simulink model "UltimoLazoAbiertoCompleto"  (R2023b)
settings: Solver=VariableStepAuto  StartTime=0.0  StopTime=2  FixedStep=0.0005  MaxStep=1e-3  RelTol=1e-3
undefined symbols (not defined in the file or in its folder): alfa, beq, Cts, ee_sli_rtmsupport, g, gcbh, id0, io0, iq0, Jeq, kl, lambda_m, Ld, Lls, Lq, Pp, r, Rs, Rts_amb, tita0, Ts0, wm0
libraries: SignalEditorBlockLib x3, eeTransforms x1, dspsigops x1, spsabctoAlphaBetaZeroLib x1
settings Model: Creator=Gustavo  LastModifiedBy=Gustavo

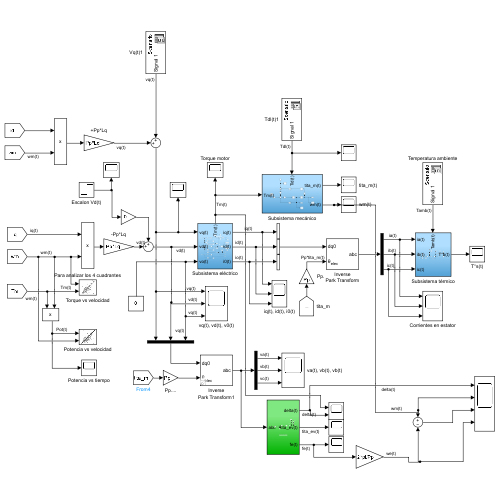
[thumbnail: Simulink's stored preview of the top-level diagram]
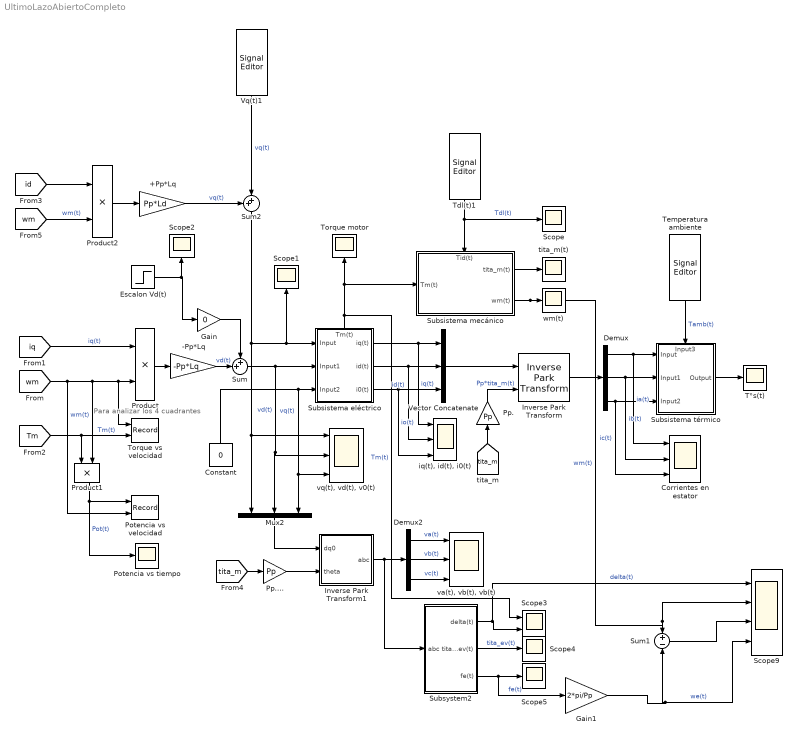
== system UltimoLazoAbiertoCompleto ==
  note: Para analizar los 4 cuadrantes
  +Pp*Lq : Gain  Gain=Pp*Ld
  -Pp*Lq : Gain  Gain=-Pp*Lq
  Constant : Constant  Value=0
  Corrientes en estator : Scope  NumInputPorts=3
  Demux : Demux  Outputs=3
  Demux2 : Demux  Outputs=3
  Escalon Vd(t) : Step  Time=0.5  After=+1.9596  SampleTime=0
  Gain : Gain  Gain=0
  Gain1 : Gain  Gain=2*pi/Pp
  Inverse Park Transform : eeTransforms/Inverse Park Transform  AxisAlignment=Q-axis  PowerInvariant=off
      settings: LibrarySourceBlock=|
      | ee_sl_lib/Mathematical
      | Transforms/Inverse
      | Park Transform
  Inverse Park Transform1 : Subsystem  AncestorBlock=|  LoadFcn=ee_sli_rtmsupport( 'loadfcn', gcbh );  mask(Inverse Park Transform){AxisAlignment=Q-axis, PowerInvariant=off}
      | ee_sl_lib/Mathematical
      | Transforms/Inverse
      | Park Transform
      mask prompts: AxisAlignment "physmod:ee:library:comments:control:eeTransforms:PhaseaAxisAlignment_MP"; PowerInvariant "physmod:ee:library:comments:control:eeTransforms:PowerInvariant_MP"
      mask help: physmod:ee:library:comments:control:eeTransforms:InverseParkTransform_MD
      mask init:
      | if PowerInvariant==0
      |     K1 = 1;
      |     K2 = 1;
      | else
      |     K1 = 1/sqrt(2);
      |     K2 = sqrt(2/3);
      | end
      | 
      | switch AxisAlignment
      |     case 'Q-axis'
      |         Offset = 0;
      |     case 'D-axis'
      |         Offset = pi/2;
      |     otherwise
      | end
      settings: CopyFcn=ee_sli_rtmsupport( 'copyfcn', gcbh );  DeleteFcn=ee_sli_rtmsupport( 'deletefcn', gcbh );  ModelCloseFcn=ee_sli_rtmsupport( 'modelclosefcn', gcbh );  PostSaveFcn=ee_sli_rtmsupport( 'postsavefcn', gcbh );  PreCopyFcn=ee_sli_rtmsupport( 'precopyfcn', gcbh );  OpenFcn=ee_sli_rtmsupport( 'openfcn', gcbh );  CloseFcn=ee_sli_rtmsupport( 'closefcn', gcbh );  PreDeleteFcn=ee_sli_rtmsupport( 'predeletefcn', gcbh );
      settings: LibrarySourceBlock=|
      | ee_sl_lib/Mathematical
      | Transforms/Inverse
      | Park Transform
      mask Help: web(nesl_help(gcbh))
      mask TypeOptions AxisAlignment: physmod:ee:library:comments:control:eeTransforms:Q0x2DAxis_PV | physmod:ee:library:comments:control:eeTransforms:D0x2DAxis_PV
      mask DialogControl AxisAlignment Prompt: Phase-a axis alignment
      mask DialogControl PowerInvariant Prompt: Power invariant
      mask Display: ee.mask.drawInverseParkTransform();
  Mux2 : Mux  Inputs=3
  Potencia vs tiempo : Scope
  Potencia vs velocidad : Record  FileSettingsInternal="{\"entries\":[{\"content\":{\"excelSettings\":{\"content\":{},\"type\":\"Streamout.ExcelSettings\"}},\"type\":\"Streamout.FileSettingStorage\",\"uuid\":\"\"}],\"packageUris\":[\"http:\\/\\/schema.mathworks.com\\/mf0\\/streamout_blocks\\/R2020a\"],\"version\":\"1.0\"}"  Layout=[1 1]  SignalsInternal="{\"entries\":[{\"content\":{\"signals\":[{\"content\":{\"blockPath\":[],\"dimensions\":[1],\"domain\":\"\",\"lineColor\":\"#139fff\",\"port\":1,\"signalID\":16,\"signalName\":\"Pot(t)\"},\"type\":\"RecordBlkView.Signal\",\"uuid\":\"\"},{\"content\":{\"blockPath\":[],\"dimensions\":[1],\"domain\":\"\",\"lineColor\":\"#ff6929\",\"port\":2,\"signalID\":19,\"signalName\":\"wm(t)\"},\"type\":\"RecordBlkView.Signal\",\"uuid\":\"\"}]},\"type\":\"RecordBlkView.InputSignals\",\"uuid\":\"\"}],\"packageUris\":[\"http:\\/\\/schema.mathworks.com\\/mf0\\/streamout_blocks\\/R2020a\"],\"version\":\"1.0\"}"  VisualizationBindings="{\"xyplotplugin\":{\"info\":[{\"series\":[],\"subplotID\":1}]}}"  CompatibilityTag=XY
  Pp. : Gain  Gain=Pp
  Pp.... : Gain  Gain=Pp
  Product : Product
  Product1 : Product
  Product2 : Product
  Scope{,1..2,4..5} (5 alike) : Scope
  Scope3 : Scope  NumInputPorts=2
  Scope9 : Scope  NumInputPorts=4
  Subsistema eléctrico : Subsystem
      settings: PortSchema="{\"entries\":[{\"content\":{\"sides\":[{\"content\":{\"connectorIds\":[\"In1\",\"In2\",\"In3\"]},\"type\":\"ConnectorPlacement.EquallySpacedRectSide\",\"uuid\":\"55314de5-b6ab-4161-b15d-819ac9b3d610\"},{\"content\":{\"connectorIds\":[\"Out1\",\"Out2\",\"Out3\"],\"side\":\"RIGHT\"},\"type\":\"ConnectorPlacement.EquallySpacedRectSide\",\"uuid\":\"6d89c228-26ff-4db5-b942-5bfef0be2fde\"},{\"content\":{\"connectorIds\":[\"Out4\"],\"side\":\"TOP\"},\"type\":\"ConnectorPlacement.EquallySpacedRectSide\",\"uuid\":\"a52f3ca3-a7f6-4886-b92b-9c9e6a107711\"}]},\"type\":\"ConnectorPlacement.EquallySpacedConnector\",\"uuid\":\"22991da4-d60d-4ddc-8bfe-b68e23663f11\"}],\"packageUris\":[\"http://schema.mathworks.com/mf0/Connector/R2020b\"],\"version\":\"1.0\"}"
  Subsistema mecánico : Subsystem
      settings: PortSchema="{\"entries\":[{\"content\":{\"sides\":[{\"content\":{\"connectorIds\":[\"In1\"]},\"type\":\"ConnectorPlacement.EquallySpacedRectSide\",\"uuid\":\"50d48cc3-d7d8-4f90-8b40-173b6a350fbf\"},{\"content\":{\"connectorIds\":[\"Out1\",\"Out2\"],\"side\":\"RIGHT\"},\"type\":\"ConnectorPlacement.EquallySpacedRectSide\",\"uuid\":\"77c04a2b-04e8-45af-8dee-d1b1ab6672f9\"},{\"content\":{\"connectorIds\":[\"In2\"],\"side\":\"TOP\"},\"type\":\"ConnectorPlacement.EquallySpacedRectSide\",\"uuid\":\"9aba66dd-f9d4-41a7-8e04-ce0a031192e2\"}]},\"type\":\"ConnectorPlacement.EquallySpacedConnector\",\"uuid\":\"47c09da0-37f3-4a5d-8fce-2546d5511531\"}],\"packageUris\":[\"http://schema.mathworks.com/mf0/Connector/R2020b\"],\"version\":\"1.0\"}"
  Subsistema térmico : Subsystem
      settings: PortSchema="{\"entries\":[{\"content\":{\"sides\":[{\"content\":{\"connectorIds\":[\"In1\",\"In2\",\"In3\"]},\"type\":\"ConnectorPlacement.EquallySpacedRectSide\",\"uuid\":\"499bb5e3-da94-498d-be5e-1974ba0b4a58\"},{\"content\":{\"connectorIds\":[\"Out1\"],\"side\":\"RIGHT\"},\"type\":\"ConnectorPlacement.EquallySpacedRectSide\",\"uuid\":\"13ea5dea-e51e-4770-b579-88e3e6e50884\"},{\"content\":{\"connectorIds\":[\"In4\"],\"side\":\"TOP\"},\"type\":\"ConnectorPlacement.EquallySpacedRectSide\",\"uuid\":\"72517ed1-a98f-428e-86e2-c370e237c602\"}]},\"type\":\"ConnectorPlacement.EquallySpacedConnector\",\"uuid\":\"7e0eda24-12d6-49d0-ad1f-024c88e78140\"}],\"packageUris\":[\"http://schema.mathworks.com/mf0/Connector/R2020b\"],\"version\":\"1.0\"}"
  Subsystem2 : Subsystem
  Sum : Sum  Inputs=++|
  Sum1 : Sum  Inputs=+|-
  Sum2 : Sum  Inputs=++|
  Tdl(t)1 : SignalEditorBlockLib/Signal Editor  FileName=SeñalTlEstadoInterno.mat  ActiveScenario=Scenario  ActiveSignal=Signal 1  IsBus=off  OutputBusObjectStr=Bus: BusObject  SampleTime=0  Interpolate=off  ZeroCross=off  OutputAfterFinalValue=Setting to zero  Unit=inherit  PreserveSignalName=on  ApplySigPropsToAllScenarios=on  ApplySigPropsToAllSignals=off
  Temperatura ambiente : SignalEditorBlockLib/Signal Editor  FileName=Temperatura ambiente Tamb(t).mat  ActiveScenario=Scenario  ActiveSignal=Signal 1  IsBus=off  OutputBusObjectStr=Bus: BusObject  SampleTime=0  ZeroCross=off  OutputAfterFinalValue=Setting to zero  Unit=inherit  PreserveSignalName=on  ApplySigPropsToAllScenarios=on  ApplySigPropsToAllSignals=off
  Torque motor : Scope
  Torque vs velocidad : Record  FileSettingsInternal="{\"entries\":[{\"content\":{\"excelSettings\":{\"content\":{},\"type\":\"Streamout.ExcelSettings\"}},\"type\":\"Streamout.FileSettingStorage\",\"uuid\":\"\"}],\"packageUris\":[\"http:\\/\\/schema.mathworks.com\\/mf0\\/streamout_blocks\\/R2020a\"],\"version\":\"1.0\"}"  Layout=[1 1]  SignalsInternal="{\"entries\":[{\"content\":{\"signals\":[{\"content\":{\"blockPath\":[],\"dimensions\":[1],\"domain\":\"\",\"lineColor\":\"#64d413\",\"port\":1,\"signalID\":8,\"signalName\":\"wm(t)\"},\"type\":\"RecordBlkView.Signal\",\"uuid\":\"\"},{\"content\":{\"blockPath\":[],\"dimensions\":[1],\"domain\":\"\",\"lineColor\":\"#ff13a6\",\"port\":2,\"signalID\":11,\"signalName\":\"Tm(t)\"},\"type\":\"RecordBlkView.Signal\",\"uuid\":\"\"}]},\"type\":\"RecordBlkView.InputSignals\",\"uuid\":\"\"}],\"packageUris\":[\"http:\\/\\/schema.mathworks.com\\/mf0\\/streamout_blocks\\/R2020a\"],\"version\":\"1.0\"}"  VisualizationBindings="{\"xyplotplugin\":{\"info\":[{\"series\":[],\"subplotID\":1}]}}"  CompatibilityTag=XY
  T°s(t) : Scope
  Vector Concatenate : Concatenate  NumInputs=3
  Vq(t)1 : SignalEditorBlockLib/Signal Editor  FileName=SeñalVQestadoInterno.mat  ActiveScenario=Scenario  ActiveSignal=Signal 1  IsBus=off  OutputBusObjectStr=Bus: BusObject  SampleTime=0  Interpolate=off  ZeroCross=off  OutputAfterFinalValue=Setting to zero  Unit=inherit  PreserveSignalName=on  ApplySigPropsToAllScenarios=on  ApplySigPropsToAllSignals=off
  "iq(t), id(t), i0(t)" : Scope  NumInputPorts=3
  tita_m(t) : Scope
  "va(t), vb(t), vb(t)" : Scope  NumInputPorts=3
  "vq(t), vd(t), v0(t)" : Scope  NumInputPorts=3
  wm(t) : Scope
  wires:
  Tdl(t)1/1 -> Subsistema mecánico/2(Tid(t)), Scope/1  "Tdl(t)"
  Subsistema eléctrico/4(Tm(t)) -> Scope3/1, Subsistema mecánico/1(Tm(t)), Torque motor/1  "Tm(t)"
  Temperatura ambiente/1 -> Subsistema térmico/4(Input3)  "Tamb(t)"
  Subsistema térmico/1(Output) -> T°s(t)/1
  Subsistema eléctrico/2(id(t)) -> "iq(t), id(t), i0(t)"/2, Vector Concatenate/2  "id(t)"
  Subsistema eléctrico/1(iq(t)) -> "iq(t), id(t), i0(t)"/1, Vector Concatenate/1  "iq(t)"
  Demux/2 -> Subsistema térmico/2(Input1), Corrientes en estator/2  "ib(t)"
  Inverse Park Transform/1 -> Demux/1
  Pp./1 -> Inverse Park Transform/2  "Pp*tita_m(t)"
  Subsistema eléctrico/3(i0(t)) -> "iq(t), id(t), i0(t)"/3, Vector Concatenate/3  "io(t)"
  [tita_m] -> Pp./1
  Vector Concatenate/1 -> Inverse Park Transform/1
  Demux/3 -> Subsistema térmico/3(Input2), Corrientes en estator/3  "ic(t)"
  Demux/1 -> Subsistema térmico/1(Input), Corrientes en estator/1  "ia(t)"
  Subsistema mecánico/2(wm(t)) -> Sum1/1, Scope9/2, wm(t)/1  "wm(t)"
  Subsistema mecánico/1(tita_m(t)) -> tita_m(t)/1
  [iq] -> Product/1  "iq(t)"
  Product/1 -> -Pp*Lq/1
  [wm] -> Torque vs velocidad/1, Product/2, Product1/2, Potencia vs velocidad/2  "wm(t)"
  Constant/1 -> Subsistema eléctrico/3(Input2), "vq(t), vd(t), v0(t)"/3, Mux2/3  "vq(t)"
  Inverse Park Transform1/1(abc) -> Subsystem2/1(abc), Demux2/1
  Demux2/1 -> "va(t), vb(t), vb(t)"/1  "va(t)"
  Demux2/3 -> "va(t), vb(t), vb(t)"/3  "vc(t)"
  Demux2/2 -> "va(t), vb(t), vb(t)"/2  "vb(t)"
  [tita_m] -> Pp..../1
  Pp..../1 -> Inverse Park Transform1/2(theta)
  Mux2/1 -> Inverse Park Transform1/1(dq0)
  [Tm] -> Torque vs velocidad/2, Product1/1  "Tm(t)"
  Product1/1 -> Potencia vs tiempo/1, Potencia vs velocidad/1  "Pot(t)"
  Escalon Vd(t)/1 -> Gain/1, Scope2/1
  -Pp*Lq/1 -> Sum/2  "vd(t)"
  Sum/1 -> Subsistema eléctrico/2(Input1), Mux2/2, "vq(t), vd(t), v0(t)"/2  "vd(t)"
  Gain/1 -> Sum/1
  Subsystem2/1(delta(t)) -> Scope9/1, Scope3/2  "delta(t)"
  Subsystem2/2(tita_ev(t)) -> Scope4/1  "tita_ev(t)"
  Subsystem2/3(fe(t)) -> Gain1/1, Scope5/1  "fe(t)"
  Gain1/1 -> Sum1/2, Scope9/4  "we(t)"
  Sum1/1 -> Scope9/3
  Vq(t)1/1 -> Sum2/2  "vq(t)"
  [wm] -> Product2/2  "wm(t)"
  [id] -> Product2/1
  Product2/1 -> +Pp*Lq/1
  +Pp*Lq/1 -> Sum2/1  "vq(t)"
  Sum2/1 -> "vq(t), vd(t), v0(t)"/1, Mux2/1, Scope1/1, Subsistema eléctrico/1(Input)

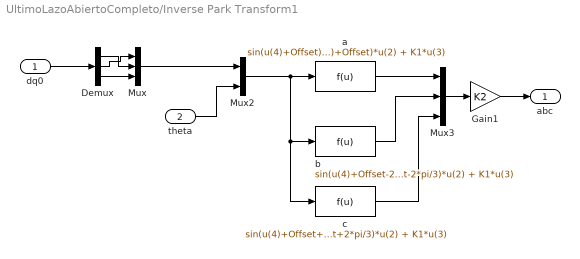
== system UltimoLazoAbiertoCompleto/Inverse Park Transform1 ==
  dq0 : Inport
  theta : Inport  Port=2
  Demux : Demux  Outputs=3
  Gain1 : Gain  Gain=K2
  Mux : Mux  Inputs=3
  Mux2 : Mux  Inputs=2
  Mux3 : Mux  Inputs=3
  a : Fcn  Expr=sin(u(4)+Offset)*u(1) + cos(u(4)+Offset)*u(2) + K1*u(3)
  b : Fcn  Expr=sin(u(4)+Offset-2*pi/3)*u(1) + cos(u(4)+Offset-2*pi/3)*u(2) + K1*u(3)
  c : Fcn  Expr=sin(u(4)+Offset+2*pi/3)*u(1) + cos(u(4)+Offset+2*pi/3)*u(2) + K1*u(3)
  abc : Outport  VectorParamsAs1DForOutWhenUnconnected=off
  wires:
  a/1 -> Mux3/1
  Mux3/1 -> Gain1/1
  Mux2/1 -> a/1, c/1, b/1
  theta/1 -> Mux2/2
  c/1 -> Mux3/3
  Gain1/1 -> abc/1
  b/1 -> Mux3/2
  Demux/2 -> Mux/1
  Demux/1 -> Mux/2
  Demux/3 -> Mux/3
  dq0/1 -> Demux/1
  Mux/1 -> Mux2/1

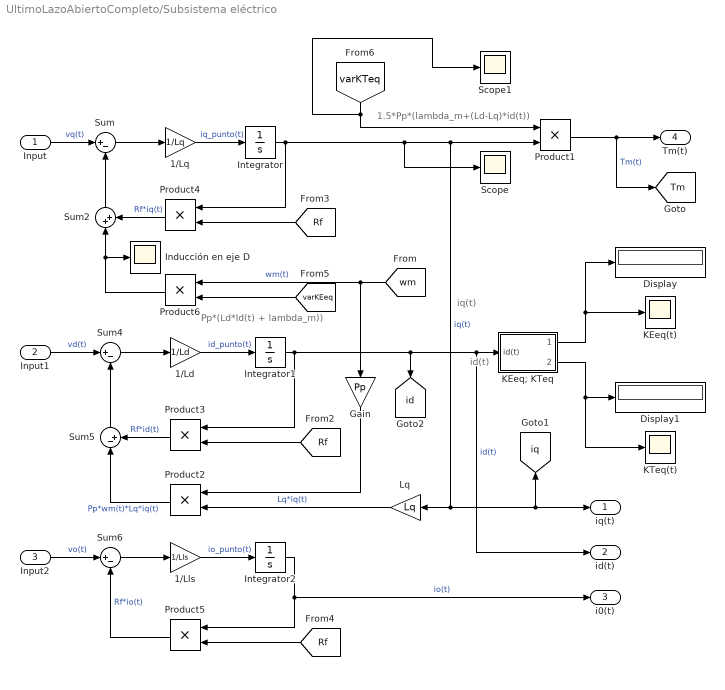
== system UltimoLazoAbiertoCompleto/Subsistema eléctrico ==
  note: 1.5*Pp*(lambda_m+(Ld-Lq)*id(t))
  note: iq(t)
  note: Pp*(Ld*Id(t) + lambda_m))
  note: id(t)
  Input : Inport
  Input1 : Inport  Port=2
  Input2 : Inport  Port=3
  1/Ld : Gain  Gain=1/Ld
  1/Lls : Gain  Gain=1/Lls
  1/Lq : Gain  Gain=1/Lq
  Display : Display
  Display1 : Display
  Gain : Gain  Gain=Pp
  Inducción en eje D : Scope
  Integrator : Integrator  InitialCondition=iq0
  Integrator1 : Integrator  InitialCondition=id0
  Integrator2 : Integrator  InitialCondition=io0
  KEeq(t) : Scope
  KEeq; KTeq : Subsystem
  KTeq(t) : Scope
  Lq : Gain  Gain=Lq
  Product{1..6} (6 alike) : Product
  Scope : Scope
  Scope1 : Scope
  Sum : Sum  Inputs=|+-
  Sum2 : Sum  Inputs=|++
  Sum4 : Sum  Inputs=|+-
  Sum5 : Sum  Inputs=|-+
  Sum6 : Sum  Inputs=|+-
  iq(t) : Outport
  id(t) : Outport  Port=2
  i0(t) : Outport  Port=3
  Tm(t) : Outport  Port=4
  tag scope: Tm=global, id=global, iq=global
  wires:
  Sum4/1 -> 1/Ld/1
  Input/1 -> Sum/1  "vq(t)"
  Integrator/1 -> Product4/1, Scope/1, Product1/2, iq(t)/1, [iq], Lq/1  "iq(t)"
  Product4/1 -> Sum2/2  "Rf*iq(t)"
  Lq/1 -> Product2/2  "Lq*iq(t)"
  Sum/1 -> 1/Lq/1
  Sum2/1 -> Sum/2
  Input2/1 -> Sum6/1  "vo(t)"
  1/Ld/1 -> Integrator1/1  "id_punto(t)"
  1/Lls/1 -> Integrator2/1  "io_punto(t)"
  Sum5/1 -> Sum4/2
  Product3/1 -> Sum5/2  "Rf*id(t)"
  Integrator1/1 -> Product3/1, [id], KEeq; KTeq/1(id(t)), id(t)/1  "id(t)"
  Integrator2/1 -> Product5/1, i0(t)/1  "io(t)"
  Input1/1 -> Sum4/1  "vd(t)"
  Product6/1 -> Inducción en eje D/1, Sum2/1
  Product5/1 -> Sum6/2  "Rf*io(t)"
  Product2/1 -> Sum5/1  "Pp*wm(t)*Lq*iq(t)"
  1/Lq/1 -> Integrator/1  "iq_punto(t)"
  Sum6/1 -> 1/Lls/1
  [wm] -> Product6/1, Gain/1  "wm(t)"
  Product1/1 -> Tm(t)/1, [Tm]  "Tm(t)"
  [Rf] -> Product3/2
  [Rf] -> Product4/2
  [Rf] -> Product5/2
  KEeq; KTeq/2(KTeq(t)) -> KTeq(t)/1, Display1/1
  KEeq; KTeq/1(KEeq(t)) -> KEeq(t)/1, Display/1
  [varKEeq] -> Product6/2
  Gain/1 -> Product2/1
  [varKTeq] -> Scope1/1, Product1/1

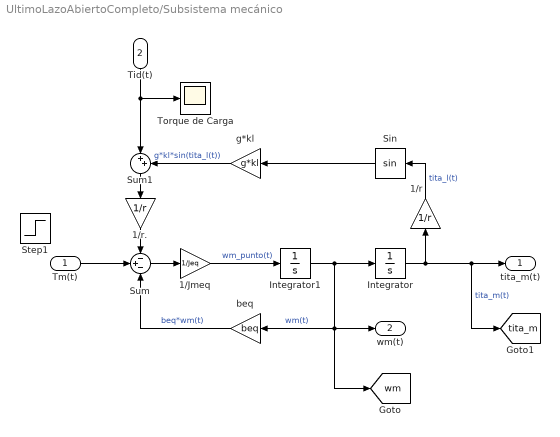
== system UltimoLazoAbiertoCompleto/Subsistema mecánico ==
  Tm(t) : Inport
  Tid(t) : Inport  Port=2
  1/Jmeq : Gain  Gain=1/Jeq
  1/r : Gain  Gain=1/r
  1/r. : Gain  Gain=1/r
  Integrator : Integrator  InitialCondition=tita0
  Integrator1 : Integrator  InitialCondition=wm0
  Sin : Trigonometry
  Step1 : Step  After=3  SampleTime=0
  Sum : Sum  Inputs=-+-
  Sum1 : Sum  Inputs=|++
  Torque de Carga : Scope
  beq : Gain  Gain=beq
  g*kl : Gain  Gain=g*kl
  tita_m(t) : Outport
  wm(t) : Outport  Port=2
  tag scope: tita_m=global, wm=global
  wires:
  Integrator/1 -> [tita_m], tita_m(t)/1, 1/r/1  "tita_m(t)"
  Integrator1/1 -> wm(t)/1, [wm], beq/1, Integrator/1  "wm(t)"
  1/r/1 -> Sin/1  "tita_l(t)"
  Sin/1 -> g*kl/1
  Sum/1 -> 1/Jmeq/1
  1/Jmeq/1 -> Integrator1/1  "wm_punto(t)"
  beq/1 -> Sum/3  "beq*wm(t)"
  Tm(t)/1 -> Sum/2
  Tid(t)/1 -> Sum1/1, Torque de Carga/1
  g*kl/1 -> Sum1/2  "g*kl*sin(tita_l(t))"
  Sum1/1 -> 1/r./1
  1/r./1 -> Sum/1

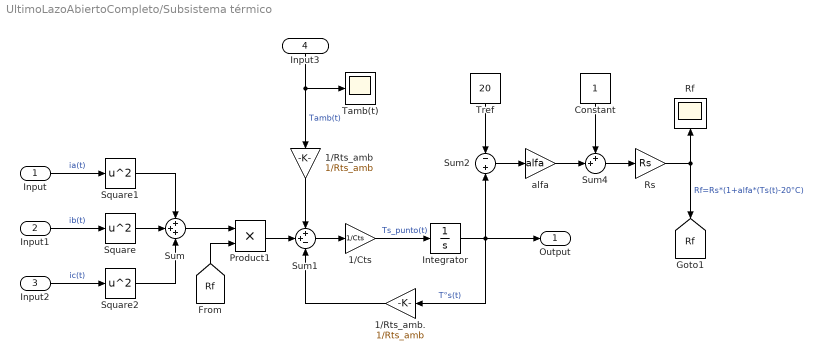
== system UltimoLazoAbiertoCompleto/Subsistema térmico ==
  Input : Inport
  Input1 : Inport  Port=2
  Input2 : Inport  Port=3
  Input3 : Inport  Port=4
  1/Cts : Gain  Gain=1/Cts
  1/Rts_amb : Gain  Gain=1/Rts_amb
  1/Rts_amb. : Gain  Gain=1/Rts_amb
  Constant : Constant
  Integrator : Integrator  InitialCondition=Ts0
  Product1 : Product
  Rf : Scope
  Rs : Gain  Gain=Rs
  Square : Math  Operator=square
  Square1 : Math  Operator=square
  Square2 : Math  Operator=square
  Sum : Sum  Inputs=+++
  Sum1 : Sum  Inputs=++-
  Sum2 : Sum  Inputs=-+
  Sum4 : Sum  Inputs=++|
  Tamb(t) : Scope
  Tref : Constant  Value=20
  alfa : Gain  Gain=alfa
  Output : Outport
  tag scope: Rf=global
  wires:
  1/Rts_amb/1 -> Sum1/1
  Sum1/1 -> 1/Cts/1
  Product1/1 -> Sum1/2
  Sum/1 -> Product1/1
  Integrator/1 -> Sum2/2, Output/1, 1/Rts_amb./1  "T°s(t)"
  1/Cts/1 -> Integrator/1  "Ts_punto(t)"
  1/Rts_amb./1 -> Sum1/3
  Square/1 -> Sum/2
  Square1/1 -> Sum/1
  Square2/1 -> Sum/3
  Input/1 -> Square1/1  "ia(t)"
  Input1/1 -> Square/1  "ib(t)"
  Input2/1 -> Square2/1  "ic(t)"
  Sum2/1 -> alfa/1
  Constant/1 -> Sum4/1
  alfa/1 -> Sum4/2
  Rs/1 -> [Rf], Rf/1  "Rf=Rs*(1+alfa*(Ts(t)-20°C)"
  [Rf] -> Product1/2
  Tref/1 -> Sum2/1
  Sum4/1 -> Rs/1
  Input3/1 -> 1/Rts_amb/1, Tamb(t)/1  "Tamb(t)"

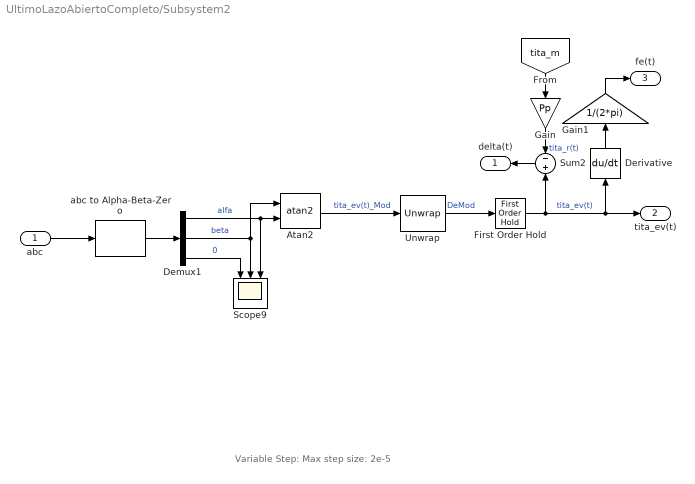
== system UltimoLazoAbiertoCompleto/Subsystem2 ==
  note: Variable Step: Max step size: 2e-5
  abc : Inport
  Atan2 : Trigonometry  Operator=atan2
  Demux1 : Demux  Outputs=3
  Derivative : Derivative
  First Order Hold : FirstOrderHold  ErrorTolerance=inf  AllowContinuousInput=on
  Gain : Gain  Gain=Pp
  Gain1 : Gain  Gain=1/(2*pi)
  Scope9 : Scope  NumInputPorts=3
  Sum2 : Sum  Inputs=-|+
  Unwrap : dspsigops/Unwrap  tol=1.2*pi  InputProcessing=Columns as channels (frame based)  running=off
  abc to Alpha-Beta-Zero : spsabctoAlphaBetaZeroLib/abc to Alpha-Beta-Zero
  delta(t) : Outport
  tita_ev(t) : Outport  Port=2
  fe(t) : Outport  Port=3
  wires:
  Demux1/1 -> Scope9/3, Atan2/2  "alfa"
  abc to Alpha-Beta-Zero/1 -> Demux1/1
  Atan2/1 -> Unwrap/1  "tita_ev(t)_Mod"
  Demux1/2 -> Scope9/2, Atan2/1  "beta"
  abc/1 -> abc to Alpha-Beta-Zero/1
  Demux1/3 -> Scope9/1  "0"
  Derivative/1 -> Gain1/1
  Gain1/1 -> fe(t)/1
  [tita_m] -> Gain/1
  Gain/1 -> Sum2/1  "tita_r(t)"
  Sum2/1 -> delta(t)/1
  Unwrap/1 -> First Order Hold/1  "DeMod"
  First Order Hold/1 -> tita_ev(t)/1, Derivative/1, Sum2/2  "tita_ev(t)"

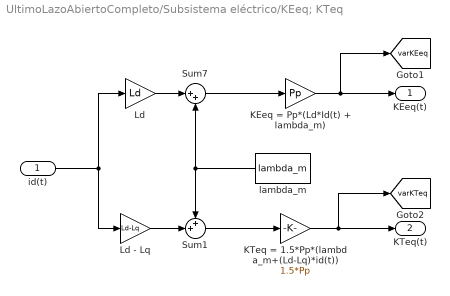
== system UltimoLazoAbiertoCompleto/Subsistema eléctrico/KEeq; KTeq ==
  id(t) : Inport
  "KEeq = Pp*(Ld*Id(t) + lambda_m) " : Gain  Gain=Pp
  "KTeq = 1.5*Pp*(lambda_m+(Ld-Lq)*id(t)) " : Gain  Gain=1.5*Pp
  Ld : Gain  Gain=Ld
  Ld - Lq : Gain  Gain=Ld-Lq
  Sum1 : Sum  Inputs=++|
  Sum7 : Sum  Inputs=|++
  lambda_m : Constant  Value=lambda_m
  KEeq(t) : Outport
  KTeq(t) : Outport  Port=2
  tag scope: varKEeq=global, varKTeq=global
  wires:
  Ld/1 -> Sum7/1
  Sum7/1 -> "KEeq = Pp*(Ld*Id(t) + lambda_m) "/1
  "KTeq = 1.5*Pp*(lambda_m+(Ld-Lq)*id(t)) "/1 -> KTeq(t)/1, [varKTeq]
  Sum1/1 -> "KTeq = 1.5*Pp*(lambda_m+(Ld-Lq)*id(t)) "/1
  id(t)/1 -> Ld/1, Ld - Lq/1
  Ld - Lq/1 -> Sum1/2
  lambda_m/1 -> Sum1/1, Sum7/2
  "KEeq = Pp*(Ld*Id(t) + lambda_m) "/1 -> [varKEeq], KEeq(t)/1
